simulink model "DigitalnputOutput"  (R2022b)
settings: Solver=FixedStepDiscrete  StartTime=0.0  StopTime=inf  FixedStep=1e-3  RelTol=1e-3
libraries: arduinolib x10, simulink x5
settings Model: Creator=tony  LastModifiedBy=tony

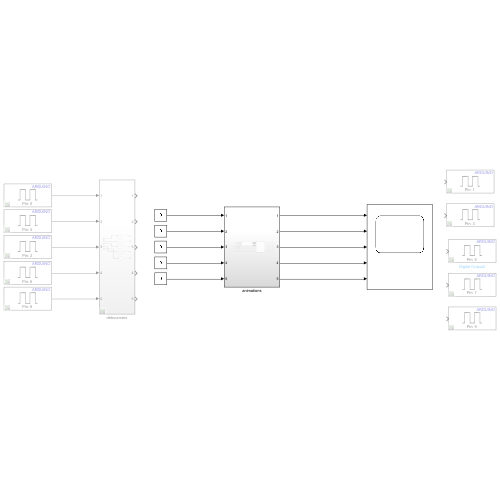
[thumbnail: Simulink's stored preview of the top-level diagram]
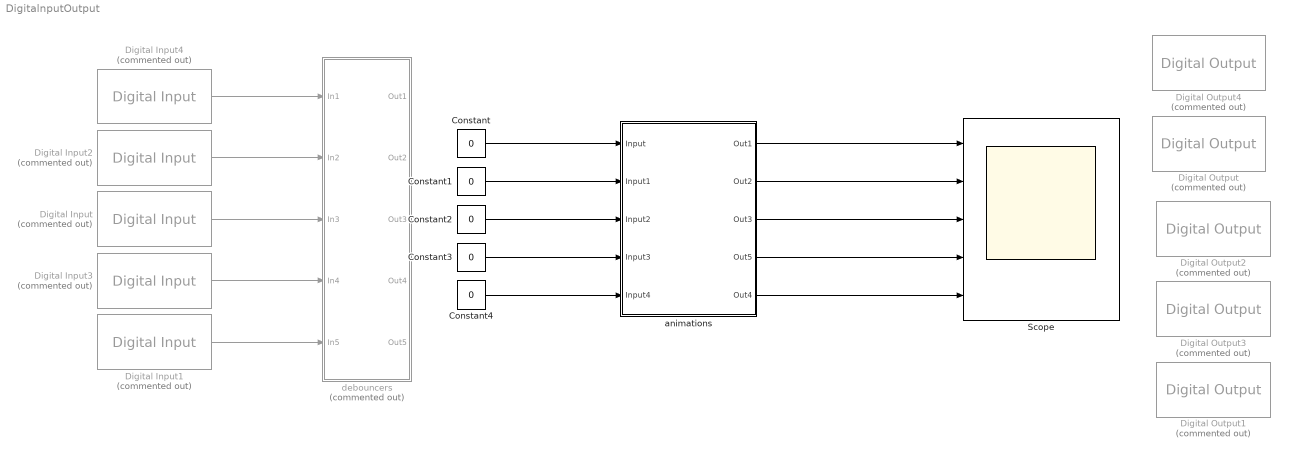
== system DigitalnputOutput ==
  Constant{,1..4} (5 alike) : Constant  Value=0
  Digital Input : arduinolib/Digital Input  Commented=on  pinNumber=2  mode=Default  Direction=input  SampleTime=0.1  blockPlatform=arduino
  Digital Input1 : arduinolib/Digital Input  Commented=on  pinNumber=8  mode=Default  Direction=input  SampleTime=0.1  blockPlatform=arduino
  Digital Input2 : arduinolib/Digital Input  Commented=on  pinNumber=4  mode=Default  Direction=input  SampleTime=0.1  blockPlatform=arduino
  Digital Input3 : arduinolib/Digital Input  Commented=on  pinNumber=6  mode=Default  Direction=input  SampleTime=0.1  blockPlatform=arduino
  Digital Input4 : arduinolib/Digital Input  Commented=on  pinNumber=0  mode=Default  Direction=input  SampleTime=0.1  blockPlatform=arduino
  Digital Output : arduinolib/Digital Output  Commented=on  pinNumber=3  Direction=output  blockPlatform=arduino
  Digital Output1 : arduinolib/Digital Output  Commented=on  pinNumber=9  Direction=output  blockPlatform=arduino
  Digital Output2 : arduinolib/Digital Output  Commented=on  pinNumber=5  Direction=output  blockPlatform=arduino
  Digital Output3 : arduinolib/Digital Output  Commented=on  pinNumber=7  Direction=output  blockPlatform=arduino
  Digital Output4 : arduinolib/Digital Output  Commented=on  pinNumber=1  Direction=output  blockPlatform=arduino
  Scope : Scope  NumInputPorts=5
  animations : Subsystem
  debouncers : Subsystem  Commented=on
  wires:
  Constant/1 -> animations/1(Input)
  Constant1/1 -> animations/2(Input1)
  Constant2/1 -> animations/3(Input2)
  Constant3/1 -> animations/4(Input3)
  Constant4/1 -> animations/5(Input4)
  animations/3(Out3) -> Scope/3
  animations/2(Out2) -> Scope/2
  animations/1(Out1) -> Scope/1
  animations/4(Out5) -> Scope/4
  animations/5(Out4) -> Scope/5
  Digital Input3/1 -> debouncers/4(In4)
  Digital Input/1 -> debouncers/3(In3)
  Digital Input1/1 -> debouncers/5(In5)
  Digital Input2/1 -> debouncers/2(In2)
  Digital Input4/1 -> debouncers/1(In1)

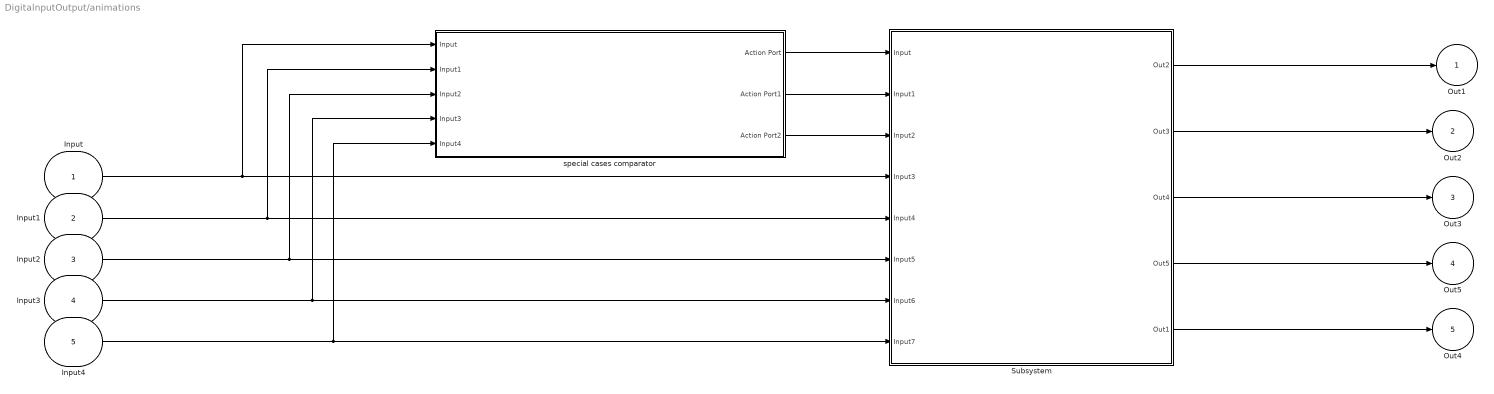
== system DigitalnputOutput/animations ==
  Input : Inport
  Input1 : Inport  Port=2
  Input2 : Inport  Port=3
  Input3 : Inport  Port=4
  Input4 : Inport  Port=5
  Subsystem : Subsystem
  special cases comparator : Subsystem
  Out1 : Outport
  Out2 : Outport  Port=2
  Out3 : Outport  Port=3
  Out5 : Outport  Port=4
  Out4 : Outport  Port=5
  wires:
  Input4/1 -> special cases comparator/5(Input4), Subsystem/8(Input7)
  Input3/1 -> special cases comparator/4(Input3), Subsystem/7(Input6)
  Input2/1 -> special cases comparator/3(Input2), Subsystem/6(Input5)
  Input1/1 -> special cases comparator/2(Input1), Subsystem/5(Input4)
  Input/1 -> special cases comparator/1(Input), Subsystem/4(Input3)
  special cases comparator/1(Action Port) -> Subsystem/1(Input)
  special cases comparator/2(Action Port1) -> Subsystem/2(Input1)
  special cases comparator/3(Action Port2) -> Subsystem/3(Input2)
  Subsystem/1(Out2) -> Out1/1
  Subsystem/2(Out3) -> Out2/1
  Subsystem/3(Out4) -> Out3/1
  Subsystem/4(Out5) -> Out5/1
  Subsystem/5(Out1) -> Out4/1

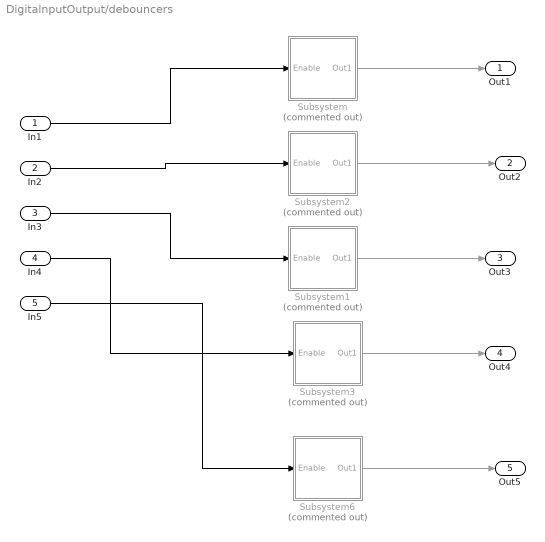
== system DigitalnputOutput/debouncers ==
  In1 : Inport
  In2 : Inport  Port=2
  In3 : Inport  Port=3
  In4 : Inport  Port=4
  In5 : Inport  Port=5
  Subsystem : Subsystem  Commented=on
  Subsystem1 : Subsystem  Commented=on
  Subsystem2 : Subsystem  Commented=on
  Subsystem3 : Subsystem  Commented=on
  Subsystem6 : Subsystem  Commented=on
  Out1 : Outport
  Out2 : Outport  Port=2
  Out3 : Outport  Port=3
  Out4 : Outport  Port=4
  Out5 : Outport  Port=5
  wires:
  In1/1 -> Subsystem/1(Enable)
  In2/1 -> Subsystem2/1(Enable)
  In3/1 -> Subsystem1/1(Enable)
  In4/1 -> Subsystem3/1(Enable)
  In5/1 -> Subsystem6/1(Enable)
  Subsystem/1(Out1) -> Out1/1
  Subsystem2/1(Out1) -> Out2/1
  Subsystem1/1(Out1) -> Out3/1
  Subsystem3/1(Out1) -> Out4/1
  Subsystem6/1(Out1) -> Out5/1

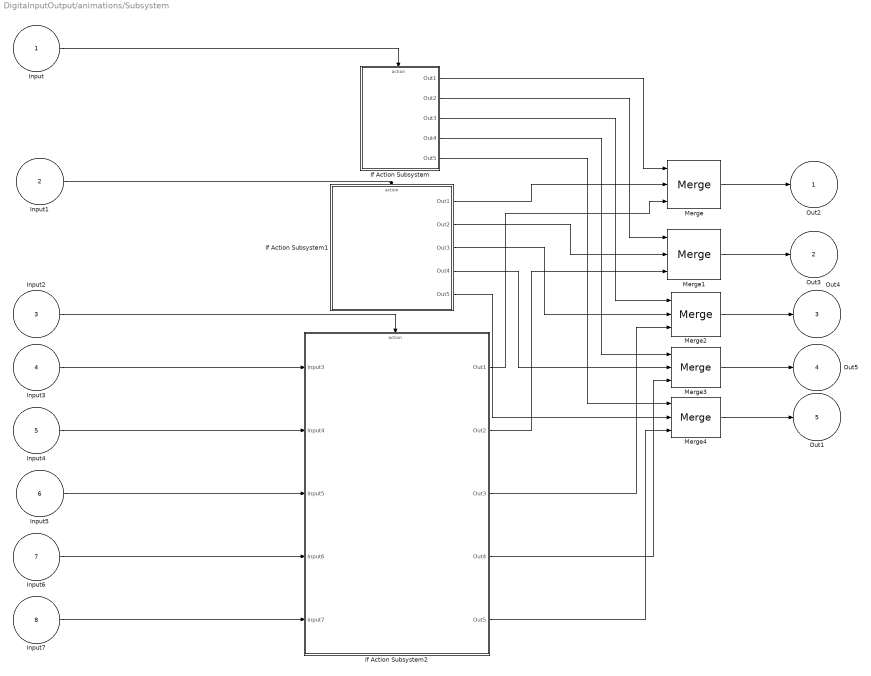
== system DigitalnputOutput/animations/Subsystem ==
  Input : Inport
  Input1 : Inport  Port=2
  Input2 : Inport  Port=3
  Input3 : Inport  Port=4
  Input4 : Inport  Port=5
  Input5 : Inport  Port=6
  Input6 : Inport  Port=7
  Input7 : Inport  Port=8
  If Action Subsystem : Subsystem  TreatAsAtomicUnit=on
  If Action Subsystem1 : Subsystem  TreatAsAtomicUnit=on
  If Action Subsystem2 : Subsystem  TreatAsAtomicUnit=on
  Merge{,1..4} (5 alike) : Merge  Inputs=3
  Out2 : Outport
  Out3 : Outport  Port=2
  Out4 : Outport  Port=3
  Out5 : Outport  Port=4
  Out1 : Outport  Port=5
  wires:
  If Action Subsystem2/5(Out5) -> Merge4/3
  If Action Subsystem1/4(Out4) -> Merge3/2
  If Action Subsystem2/1(Out1) -> Merge/3
  If Action Subsystem2/3(Out3) -> Merge2/3
  If Action Subsystem1/1(Out1) -> Merge/2
  If Action Subsystem/5(Out5) -> Merge4/1
  If Action Subsystem2/2(Out2) -> Merge1/3
  If Action Subsystem/3(Out3) -> Merge2/1
  If Action Subsystem/4(Out4) -> Merge3/1
  If Action Subsystem/1(Out1) -> Merge/1
  If Action Subsystem1/3(Out3) -> Merge2/2
  If Action Subsystem1/5(Out5) -> Merge4/2
  If Action Subsystem1/2(Out2) -> Merge1/2
  If Action Subsystem/2(Out2) -> Merge1/1
  If Action Subsystem2/4(Out4) -> Merge3/3
  Input/1 -> If Action Subsystem/Action
  Input1/1 -> If Action Subsystem1/Action
  Input2/1 -> If Action Subsystem2/Action
  Input3/1 -> If Action Subsystem2/1(Input3)
  Input4/1 -> If Action Subsystem2/2(Input4)
  Input5/1 -> If Action Subsystem2/3(Input5)
  Input6/1 -> If Action Subsystem2/4(Input6)
  Input7/1 -> If Action Subsystem2/5(Input7)
  Merge/1 -> Out2/1
  Merge1/1 -> Out3/1
  Merge2/1 -> Out4/1
  Merge3/1 -> Out5/1
  Merge4/1 -> Out1/1

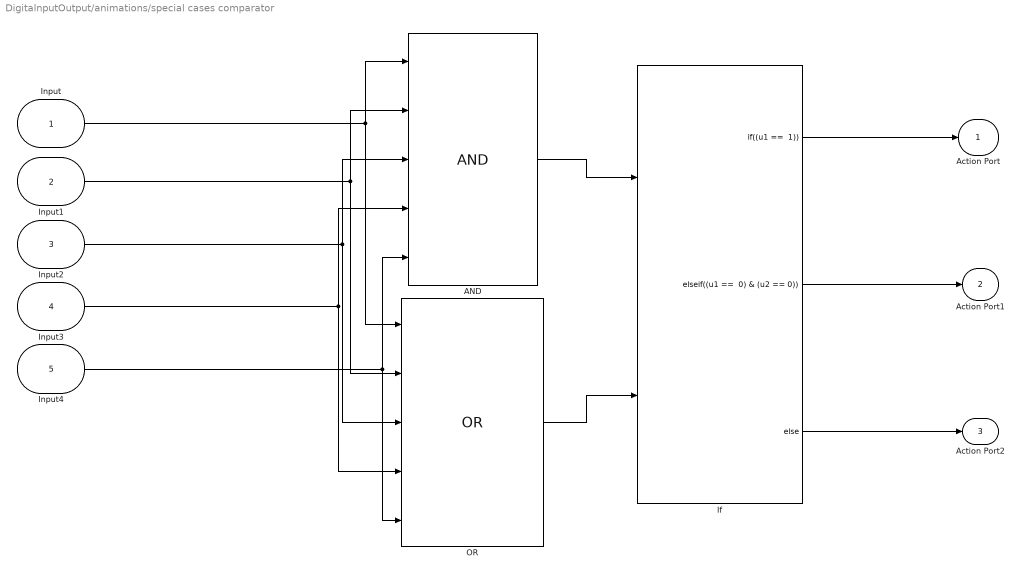
== system DigitalnputOutput/animations/special cases comparator ==
  Input : Inport
  Input1 : Inport  Port=2
  Input2 : Inport  Port=3
  Input3 : Inport  Port=4
  Input4 : Inport  Port=5
  AND : Logic  Inputs=5  IconShape=distinctive  AllPortsSameDT=off  OutDataTypeStr=boolean
  If : If  NumInputs=2  IfExpression="(u1 ==  1)"  ElseIfExpressions="(u1 ==  0) & (u2 == 0)"
  OR : Logic  Operator=OR  Inputs=5  IconShape=distinctive  AllPortsSameDT=off  OutDataTypeStr=boolean
  Action Port : Outport
  Action Port1 : Outport  Port=2
  Action Port2 : Outport  Port=3
  wires:
  Input3/1 -> OR/4, AND/4
  Input/1 -> OR/1, AND/1
  Input1/1 -> OR/2, AND/2
  Input4/1 -> AND/5, OR/5
  Input2/1 -> OR/3, AND/3
  AND/1 -> If/1
  If/2 -> Action Port1/1
  If/3 -> Action Port2/1
  If/1 -> Action Port/1
  OR/1 -> If/2

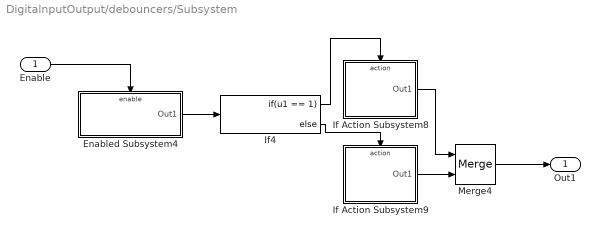
== system DigitalnputOutput/debouncers/Subsystem ==
  Enable : Inport
  Enabled Subsystem4 : Subsystem  TreatAsAtomicUnit=on
  If Action Subsystem8 : Subsystem  TreatAsAtomicUnit=on
  If Action Subsystem9 : Subsystem  TreatAsAtomicUnit=on
  If4 : If  IfExpression=u1 == 1
  Merge4 : Merge
  Out1 : Outport
  wires:
  If Action Subsystem9/1(Out1) -> Merge4/2
  Enabled Subsystem4/1(Out1) -> If4/1
  If Action Subsystem8/1(Out1) -> Merge4/1
  If4/1 -> If Action Subsystem8/Action
  Enable/1 -> Enabled Subsystem4/Enable
  Merge4/1 -> Out1/1
  If4/2 -> If Action Subsystem9/Action

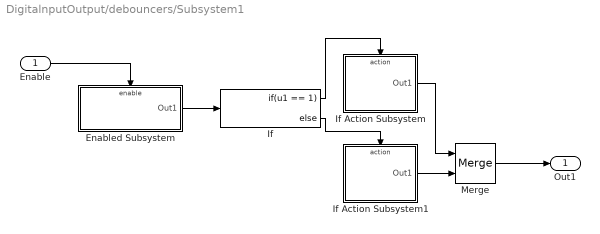
== system DigitalnputOutput/debouncers/Subsystem1 ==
  Enable : Inport
  Enabled Subsystem : Subsystem  TreatAsAtomicUnit=on
  If : If  IfExpression=u1 == 1
  If Action Subsystem : Subsystem  TreatAsAtomicUnit=on
  If Action Subsystem1 : Subsystem  TreatAsAtomicUnit=on
  Merge : Merge
  Out1 : Outport
  wires:
  Enable/1 -> Enabled Subsystem/Enable
  Enabled Subsystem/1(Out1) -> If/1
  If Action Subsystem1/1(Out1) -> Merge/2
  If/1 -> If Action Subsystem/Action
  Merge/1 -> Out1/1
  If Action Subsystem/1(Out1) -> Merge/1
  If/2 -> If Action Subsystem1/Action

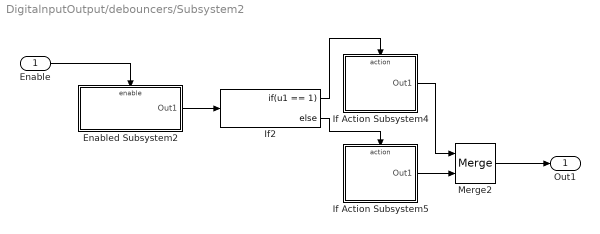
== system DigitalnputOutput/debouncers/Subsystem2 ==
  Enable : Inport
  Enabled Subsystem2 : Subsystem  TreatAsAtomicUnit=on
  If Action Subsystem4 : Subsystem  TreatAsAtomicUnit=on
  If Action Subsystem5 : Subsystem  TreatAsAtomicUnit=on
  If2 : If  IfExpression=u1 == 1
  Merge2 : Merge
  Out1 : Outport
  wires:
  If2/2 -> If Action Subsystem5/Action
  If Action Subsystem5/1(Out1) -> Merge2/2
  Enable/1 -> Enabled Subsystem2/Enable
  Enabled Subsystem2/1(Out1) -> If2/1
  If2/1 -> If Action Subsystem4/Action
  Merge2/1 -> Out1/1
  If Action Subsystem4/1(Out1) -> Merge2/1

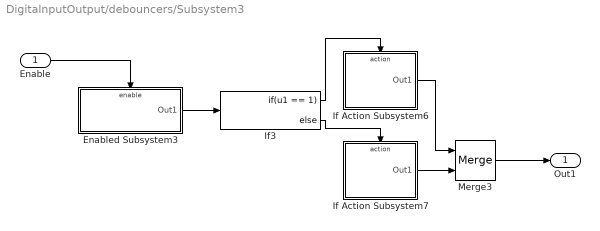
== system DigitalnputOutput/debouncers/Subsystem3 ==
  Enable : Inport
  Enabled Subsystem3 : Subsystem  TreatAsAtomicUnit=on
  If Action Subsystem6 : Subsystem  TreatAsAtomicUnit=on
  If Action Subsystem7 : Subsystem  TreatAsAtomicUnit=on
  If3 : If  IfExpression=u1 == 1
  Merge3 : Merge
  Out1 : Outport
  wires:
  Merge3/1 -> Out1/1
  If Action Subsystem6/1(Out1) -> Merge3/1
  If Action Subsystem7/1(Out1) -> Merge3/2
  If3/2 -> If Action Subsystem7/Action
  If3/1 -> If Action Subsystem6/Action
  Enable/1 -> Enabled Subsystem3/Enable
  Enabled Subsystem3/1(Out1) -> If3/1

== system DigitalnputOutput/debouncers/Subsystem6 ==
  Enable : Inport
  Enabled Subsystem1 : Subsystem  TreatAsAtomicUnit=on
  If Action Subsystem2 : Subsystem  TreatAsAtomicUnit=on
  If Action Subsystem3 : Subsystem  TreatAsAtomicUnit=on
  If1 : If  IfExpression=u1 == 1
  Merge1 : Merge
  Out1 : Outport
  wires:
  If1/1 -> If Action Subsystem2/Action
  Enable/1 -> Enabled Subsystem1/Enable
  If Action Subsystem2/1(Out1) -> Merge1/1
  If Action Subsystem3/1(Out1) -> Merge1/2
  If1/2 -> If Action Subsystem3/Action
  Enabled Subsystem1/1(Out1) -> If1/1
  Merge1/1 -> Out1/1

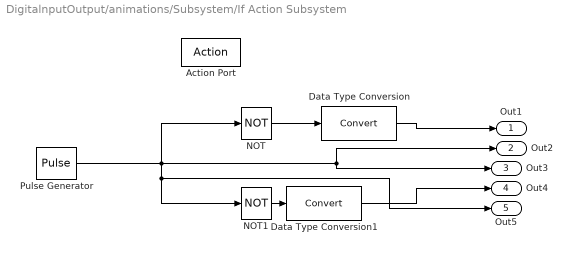
== system DigitalnputOutput/animations/Subsystem/If Action Subsystem ==
  Action Port : ActionPort  ActionPortLabel="if((u1 ==  1))"
  Data Type Conversion : DataTypeConversion  SaturateOnIntegerOverflow=off  RndMeth=Floor
  Data Type Conversion1 : DataTypeConversion  SaturateOnIntegerOverflow=off  RndMeth=Floor
  NOT : Logic  Operator=NOT  IconShape=distinctive  AllPortsSameDT=off  OutDataTypeStr=fixdt(1,16)
  NOT1 : Logic  Operator=NOT  IconShape=distinctive  AllPortsSameDT=off  OutDataTypeStr=fixdt(1,16)
  Pulse Generator : DiscretePulseGenerator  PulseType=Time based  Period=10  PulseWidth=50
  Out1 : Outport
  Out2 : Outport  Port=2
  Out3 : Outport  Port=3
  Out4 : Outport  Port=4
  Out5 : Outport  Port=5
  wires:
  Pulse Generator/1 -> Out3/1, Out2/1, Out5/1, NOT1/1, NOT/1
  NOT/1 -> Data Type Conversion/1
  Data Type Conversion/1 -> Out1/1
  NOT1/1 -> Data Type Conversion1/1
  Data Type Conversion1/1 -> Out4/1

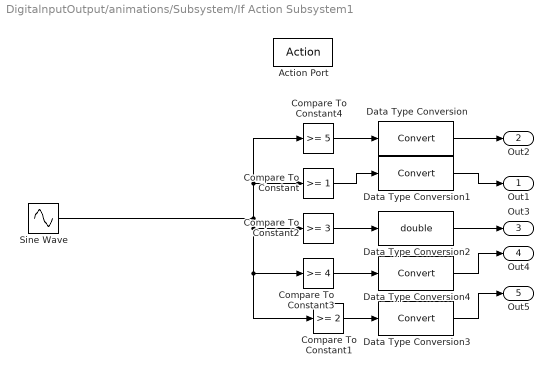
== system DigitalnputOutput/animations/Subsystem/If Action Subsystem1 ==
  Action Port : ActionPort  ActionPortLabel="elseif((u1 ==  0) & (u2 == 0))"
  Compare To Constant : simulink/Logic and Bit Operations/Compare To Constant  relop=>=  const=1  OutDataTypeStr=uint8
  Compare To Constant1 : simulink/Logic and Bit Operations/Compare To Constant  relop=>=  const=2  OutDataTypeStr=uint8
  Compare To Constant2 : simulink/Logic and Bit Operations/Compare To Constant  relop=>=  const=3  OutDataTypeStr=uint8
  Compare To Constant3 : simulink/Logic and Bit Operations/Compare To Constant  relop=>=  const=4  OutDataTypeStr=uint8
  Compare To Constant4 : simulink/Logic and Bit Operations/Compare To Constant  relop=>=  const=5  OutDataTypeStr=uint8
  Data Type Conversion{,1,3..4} (4 alike) : DataTypeConversion  SaturateOnIntegerOverflow=off  RndMeth=Floor
  Data Type Conversion2 : DataTypeConversion  OutDataTypeStr=double  SaturateOnIntegerOverflow=off  RndMeth=Floor
  Sine Wave : Sin  Amplitude=5  Frequency=0.01
  Out1 : Outport
  Out2 : Outport  Port=2
  Out3 : Outport  Port=3
  Out4 : Outport  Port=4
  Out5 : Outport  Port=5
  wires:
  Compare To Constant3/1 -> Data Type Conversion4/1
  Compare To Constant2/1 -> Data Type Conversion2/1
  Compare To Constant/1 -> Data Type Conversion1/1
  Sine Wave/1 -> Compare To Constant1/1, Compare To Constant3/1, Compare To Constant2/1, Compare To Constant/1, Compare To Constant4/1
  Compare To Constant4/1 -> Data Type Conversion/1
  Data Type Conversion/1 -> Out2/1
  Data Type Conversion1/1 -> Out1/1
  Data Type Conversion2/1 -> Out3/1
  Data Type Conversion4/1 -> Out4/1
  Compare To Constant1/1 -> Data Type Conversion3/1
  Data Type Conversion3/1 -> Out5/1

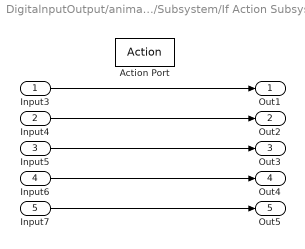
== system DigitalnputOutput/animations/Subsystem/If Action Subsystem2 ==
  Input3 : Inport
  Input4 : Inport  Port=2
  Input5 : Inport  Port=3
  Input6 : Inport  Port=4
  Input7 : Inport  Port=5
  Action Port : ActionPort  ActionPortLabel=else
  Out1 : Outport
  Out2 : Outport  Port=2
  Out3 : Outport  Port=3
  Out4 : Outport  Port=4
  Out5 : Outport  Port=5
  wires:
  Input3/1 -> Out1/1
  Input4/1 -> Out2/1
  Input5/1 -> Out3/1
  Input6/1 -> Out4/1
  Input7/1 -> Out5/1

== system DigitalnputOutput/debouncers/Subsystem/Enabled Subsystem4 ==
  Enable : EnablePort  StatesWhenEnabling=reset
  Add : Sum
  Constant : Constant
  Unit Delay : UnitDelay  SampleTime=-1  HasFrameUpgradeWarning=on
  Out1 : Outport
  wires:
  Constant/1 -> Add/1
  Unit Delay/1 -> Add/2
  Add/1 -> Out1/1, Unit Delay/1

== system DigitalnputOutput/debouncers/Subsystem/If Action Subsystem8 ==
  Action Port : ActionPort
  Constant : Constant
  Out1 : Outport
  wires:
  Constant/1 -> Out1/1

== system DigitalnputOutput/debouncers/Subsystem/If Action Subsystem9 ==
  Action Port : ActionPort
  Constant : Constant  Value=0
  Out1 : Outport
  wires:
  Constant/1 -> Out1/1

== system DigitalnputOutput/debouncers/Subsystem1/Enabled Subsystem ==
  Enable : EnablePort  StatesWhenEnabling=reset
  Add : Sum
  Constant : Constant
  Unit Delay : UnitDelay  SampleTime=-1  HasFrameUpgradeWarning=on
  Out1 : Outport
  wires:
  Add/1 -> Unit Delay/1, Out1/1
  Unit Delay/1 -> Add/2
  Constant/1 -> Add/1

== system DigitalnputOutput/debouncers/Subsystem1/If Action Subsystem ==
  Action Port : ActionPort
  Constant : Constant
  Out1 : Outport
  wires:
  Constant/1 -> Out1/1

== system DigitalnputOutput/debouncers/Subsystem1/If Action Subsystem1 ==
  Action Port : ActionPort
  Constant : Constant  Value=0
  Out1 : Outport
  wires:
  Constant/1 -> Out1/1

== system DigitalnputOutput/debouncers/Subsystem2/Enabled Subsystem2 ==
  Enable : EnablePort  StatesWhenEnabling=reset
  Add : Sum
  Constant : Constant
  Unit Delay : UnitDelay  SampleTime=-1  HasFrameUpgradeWarning=on
  Out1 : Outport
  wires:
  Add/1 -> Unit Delay/1, Out1/1
  Unit Delay/1 -> Add/2
  Constant/1 -> Add/1

== system DigitalnputOutput/debouncers/Subsystem2/If Action Subsystem4 ==
  Action Port : ActionPort
  Constant : Constant
  Out1 : Outport
  wires:
  Constant/1 -> Out1/1

== system DigitalnputOutput/debouncers/Subsystem2/If Action Subsystem5 ==
  Action Port : ActionPort
  Constant : Constant  Value=0
  Out1 : Outport
  wires:
  Constant/1 -> Out1/1

== system DigitalnputOutput/debouncers/Subsystem3/Enabled Subsystem3 ==
  Enable : EnablePort  StatesWhenEnabling=reset
  Add : Sum
  Constant : Constant
  Unit Delay : UnitDelay  SampleTime=-1  HasFrameUpgradeWarning=on
  Out1 : Outport
  wires:
  Add/1 -> Unit Delay/1, Out1/1
  Unit Delay/1 -> Add/2
  Constant/1 -> Add/1

== system DigitalnputOutput/debouncers/Subsystem3/If Action Subsystem6 ==
  Action Port : ActionPort
  Constant : Constant
  Out1 : Outport
  wires:
  Constant/1 -> Out1/1

== system DigitalnputOutput/debouncers/Subsystem3/If Action Subsystem7 ==
  Action Port : ActionPort
  Constant : Constant  Value=0
  Out1 : Outport
  wires:
  Constant/1 -> Out1/1

== system DigitalnputOutput/debouncers/Subsystem6/Enabled Subsystem1 ==
  Enable : EnablePort  StatesWhenEnabling=reset
  Add : Sum
  Constant : Constant
  Unit Delay : UnitDelay  SampleTime=-1  HasFrameUpgradeWarning=on
  Out1 : Outport
  wires:
  Add/1 -> Unit Delay/1, Out1/1
  Unit Delay/1 -> Add/2
  Constant/1 -> Add/1

== system DigitalnputOutput/debouncers/Subsystem6/If Action Subsystem2 ==
  Action Port : ActionPort
  Constant : Constant
  Out1 : Outport
  wires:
  Constant/1 -> Out1/1

== system DigitalnputOutput/debouncers/Subsystem6/If Action Subsystem3 ==
  Action Port : ActionPort
  Constant : Constant  Value=0
  Out1 : Outport
  wires:
  Constant/1 -> Out1/1
